simulink model "Wyparka"  (R2022a)
settings: Solver=ode45  StartTime=0.0  StopTime=300  FixedStep=0.1  RelTol=1e-6  EnableMultiTasking=on
values from neighbouring files (symbols this model uses):
  F1 = sprob + 9.5    [generator.m]    (also in sfunkcja.m = u(5); test.m = 10)
  F2 = u(1)    [sfunkcja.m]    (also in test.m = 2)
  F200 = u(3)    [sfunkcja.m]    (also in test.m = 208)
  F3 = u(4)    [sfunkcja.m]    (also in test.m = 50)
  P100 = u(2)    [sfunkcja.m]    (also in test.m = 194.7)
  T1 = u(7)    [sfunkcja.m]    (also in test.m = 40)
  T200 = u(8)    [sfunkcja.m]    (also in test.m = 25)
  X1 = u(6)    [sfunkcja.m]    (also in test.m = 5)
libraries: slpidlib x1
settings Model: Creator=Maciek  LastModifiedBy=M
settings SolverCC: AlgebraicLoopSolver=TrustRegion
settings DataIOCC: SaveFormat=Array  SignalLoggingSaveFormat=ModelDataLogs  ReturnWorkspaceOutputs=off
settings OptimizationCC: ExpressionDepthLimit=2147483647  LifeSpan=inf
settings DebuggingCC: UnderspecifiedInitializationDetection=Classic  MergeDetectMultiDrivingBlocksExec=none  SolverPrmCheckMsg=warning  FcnCallInpInsideContextMsg=warning  UnconnectedInputMsg=warning  UnconnectedOutputMsg=warning  UnconnectedLineMsg=warning  StateNameClashWarn=warning  SFUnexpectedBacktrackingDiag=warning  SFNoUnconditionalDefaultTransitionDiag=warning  SFExecutionAtInitializationDiag=none  SFMachineParentedDataDiag=warning  ArithmeticOperatorsInVariantConditions=warning
settings HardwareCC: ProdBitPerPointer=32  ProdBitPerSizeT=32  ProdBitPerPtrDiffT=32  ProdLargestAtomicFloat=None  ProdIntDivRoundTo=Undefined  ProdEndianess=Unspecified  ProdWordSize=32  ProdHWDeviceType=32-bit Generic
settings ModelReferenceCC: PropagateSignalLabelsOutOfModel=off
settings SFSimCC: SimUseLocalCustomCode=off  CustomCodeUndefinedFunction=UseInterfaceOnly
settings RTWCC: RTWUseLocalCustomCode=off
settings CodeAppCC: StateflowObjectComments=on
settings GRTTargetCC: TargetLangStandard=C89/C90 (ANSI)  CombineOutputUpdateFcns=off  GRTInterface=on
settings ConfigComp: CovMetricSettings=dw  CovSaveCumulativeToWorkspaceVar=on  CovSaveSingleToWorkspaceVar=on  CovExternalEMLEnable=off

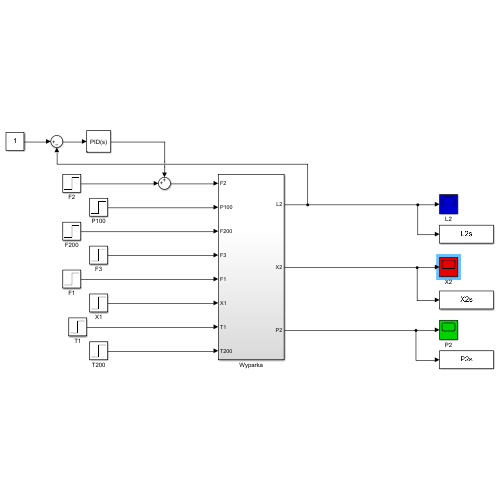
[thumbnail: Simulink's stored preview of the top-level diagram]
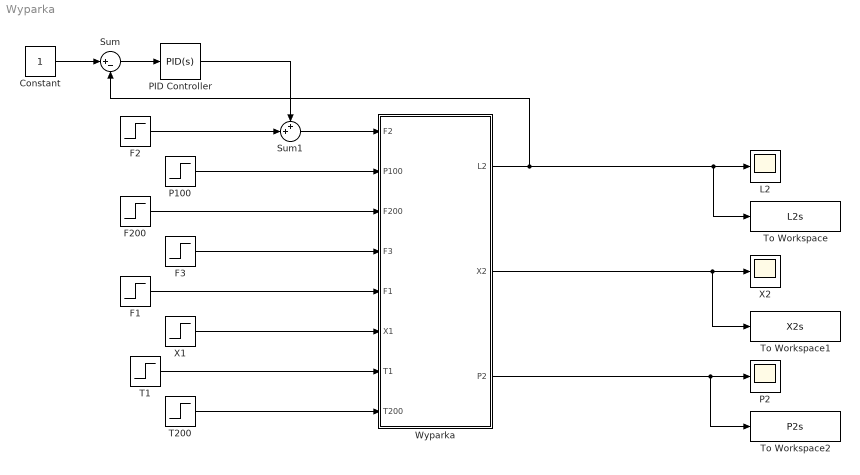
== system Wyparka ==
  Constant : Constant
  F1 : Step  Time=0  Before=F1  After=F1  SampleTime=0
  F2 : Step  Time=0  Before=F2  After=F2  SampleTime=0
  F200 : Step  Time=0  Before=F200  After=F200  SampleTime=0
  F3 : Step  Time=0  Before=F3  After=F3  SampleTime=0
  L2 : Scope
  P100 : Step  Time=0  Before=P100  After=P100  SampleTime=0
  P2 : Scope
  PID Controller : slpidlib/PID Controller  Controller=PID  Form=Parallel  TimeDomain=Continuous-time  UseExternalTs=off  SampleTime=-1  IntegratorMethod=Forward Euler  FilterMethod=Forward Euler  ControllerParametersSource=internal  P=-190.185961057962  I=-335.1597134707  UseKiTs=off  D=-3.82828237145313  N=36.46824066771  UseFilter=on  TunerSelectOption=Transfer Function Based (PID Tuner App)  InitialConditionSource=internal  InitialConditionForIntegrator=0  InitialConditionForFilter=0  DifferentiatorICPrevScaledInput=0  ExternalReset=none  TrackingMode=off  Kt=1  LimitOutput=off  SatLimitsSource=internal  UpperSaturationLimit=inf  LowerSaturationLimit=-inf  LinearizeAsGain=on  AntiWindupMode=none  Kb=1  POutMin=[]  POutMax=[]  IOutMin=[]  IOutMax=[]  DOutMin=[]  DOutMax=[]  NOutMin=[]  NOutMax=[]  SumOutMin=[]  SumOutMax=[]  SaturationOutMin=[]  SaturationOutMax=[]  PParamMin=[]  PParamMax=[]  IParamMin=[]  IParamMax=[]  DParamMin=[]  DParamMax=[]  NParamMin=[]  NParamMax=[]  KbParamMin=[]  KbParamMax=[]  KtParamMin=[]  KtParamMax=[]  KbOutMin=[]  KbOutMax=[]  KtOutMin=[]  KtOutMax=[]  IntegratorOutMin=[]  IntegratorOutMax=[]  FilterOutMin=[]  FilterOutMax=[]  SumI1OutMin=[]  SumI1OutMax=[]  SumI2OutMin=[]  SumI2OutMax=[]  SumI3OutMin=[]  SumI3OutMax=[]  SumI4OutMin=[]  SumI4OutMax=[]  SumDOutMin=[]  SumDOutMax=[]  DifferentiatorOutMin=[]  DifferentiatorOutMax=[]  FilterDiffOutCoefMin=[]  FilterDiffOutCoefMax=[]  ReciprocalOutMin=[]  ReciprocalOutMax=[]  SumDenOutMin=[]  SumDenOutMax=[]  SumNumOutMin=[]  SumNumOutMax=[]  DivideOutMin=[]  DivideOutMax=[]  UdiffTsProdOutMin=[]  UdiffTsProdOutMax=[]  NTsProdOutMin=[]  NTsProdOutMax=[]  UintegralTsProdOutMin=[]  UintegralTsProdOutMax=[]  UngainTsProdOutMin=[]  UngainTsProdOutMax=[]  IntegratorContinuousStateAttributes=''  IntegratorStateMustResolveToSignalObject=off  IntegratorRTWStateStorageClass=Auto  FilterContinuousStateAttributes=''  FilterStateMustResolveToSignalObject=off  FilterRTWStateStorageClass=Auto  ParallelPVariant=InternalParameters  IdealPVariant=Disabled  IVariant=InternalParameters  DVariant=InternalParameters  IntegratorVariant=Continuous  SatVariant=Disabled  AWVariant=Passthrough  PCopyVariant=Disabled  TRVariant=Disabled  FdbkBlocksVariant=Forward  IdealPFdbkVariant=Disabled  SatFdbkVariant=Disabled  DerivativeFilterVariant=ContFilter  NVariant=InternalParameters  NCopyVariant=Disabled  FilterICVariant=InternalICsFilter  IntegratorICVariant=InternalICs  ExternalResetVariant=Disabled  TRSumVariant=Passthrough  SumFdbkVariant=Disabled  SumVariant=Sum_PID  TsampFilterVariant=InternalTs  TsampNgainVariant=Passthrough  TsampIntegralVariant=Passthrough  ExternalSaturationOutDataTypeStr=Inherit: Same as second input  aMode=0
  Sum : Sum  Inputs=|+-
  Sum1 : Sum  Inputs=++|
  T1 : Step  Time=0  Before=T1  After=T1  SampleTime=0
  T200 : Step  Time=0  Before=T200  After=T200  SampleTime=0
  To Workspace : ToWorkspace  VariableName=L2s  SaveFormat=Structure With Time  SampleTime=-1
  To Workspace1 : ToWorkspace  VariableName=X2s  SaveFormat=Structure With Time  SampleTime=-1
  To Workspace2 : ToWorkspace  VariableName=P2s  SaveFormat=Structure With Time  SampleTime=-1
  Wyparka : Subsystem
  X1 : Step  Time=0  Before=X1  After=X1  SampleTime=0
  X2 : Scope
  wires:
  Wyparka/2(X2) -> To Workspace1/1, X2/1
  Wyparka/3(P2) -> To Workspace2/1, P2/1
  F3/1 -> Wyparka/4(F3)
  P100/1 -> Wyparka/2(P100)
  F1/1 -> Wyparka/5(F1)
  T1/1 -> Wyparka/7(T1)
  T200/1 -> Wyparka/8(T200)
  F200/1 -> Wyparka/3(F200)
  X1/1 -> Wyparka/6(X1)
  Sum/1 -> PID Controller/1
  Wyparka/1(L2) -> Sum/2, To Workspace/1, L2/1
  Constant/1 -> Sum/1
  F2/1 -> Sum1/2
  PID Controller/1 -> Sum1/1
  Sum1/1 -> Wyparka/1(F2)

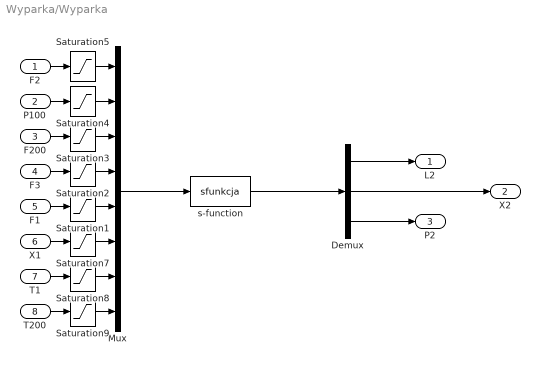
== system Wyparka/Wyparka ==
  F2 : Inport
  P100 : Inport  Port=2
  F200 : Inport  Port=3
  F3 : Inport  Port=4
  F1 : Inport  Port=5
  X1 : Inport  Port=6
  T1 : Inport  Port=7
  T200 : Inport  Port=8
  Demux : Demux  Outputs=3
  Mux : Mux  Inputs=8
  Saturation1 : Saturate  UpperLimit=20  LowerLimit=0
  Saturation2 : Saturate  UpperLimit=100  LowerLimit=0
  Saturation3 : Saturate  UpperLimit=400  LowerLimit=0
  Saturation4 : Saturate  UpperLimit=400  LowerLimit=0
  Saturation5 : Saturate  UpperLimit=4  LowerLimit=0
  Saturation7 : Saturate  UpperLimit=100  LowerLimit=0
  Saturation8 : Saturate  UpperLimit=90  LowerLimit=5
  Saturation9 : Saturate  UpperLimit=90  LowerLimit=5
  s-function : S-Function  FunctionName=sfunkcja  SFunctionDeploymentMode=off  EnableBusSupport=off
  L2 : Outport
  X2 : Outport  Port=2
  P2 : Outport  Port=3
  wires:
  s-function/1 -> Demux/1
  Mux/1 -> s-function/1
  P100/1 -> Saturation4/1
  Demux/1 -> L2/1
  F200/1 -> Saturation3/1
  Demux/2 -> X2/1
  F3/1 -> Saturation2/1
  Demux/3 -> P2/1
  F1/1 -> Saturation1/1
  X1/1 -> Saturation7/1
  T1/1 -> Saturation8/1
  T200/1 -> Saturation9/1
  F2/1 -> Saturation5/1
  Saturation1/1 -> Mux/5
  Saturation2/1 -> Mux/4
  Saturation3/1 -> Mux/3
  Saturation4/1 -> Mux/2
  Saturation5/1 -> Mux/1
  Saturation7/1 -> Mux/6
  Saturation8/1 -> Mux/7
  Saturation9/1 -> Mux/8
